simulink model "DiagramaDeBlocosDrone"  (R2014a)
settings: Solver=ode45  StartTime=0.0  StopTime=10.0  RelTol=1e-3
undefined symbols (not defined in the file): K
libraries: fuzblock x2
settings Model: Creator=ASAFE  LastModifiedBy=ASAFE

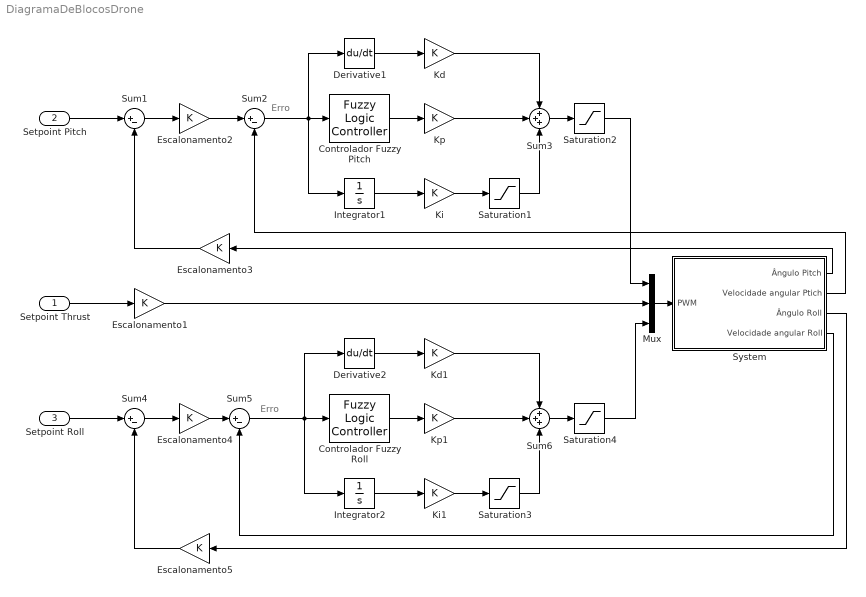
== system DiagramaDeBlocosDrone ==
  note: Erro
  note: Erro
  Setpoint Thrust : Inport
  Setpoint Pitch : Inport  Port=2
  Setpoint Roll : Inport  Port=3
  Controlador Fuzzy Pitch : fuzblock/Fuzzy Logic  Controller  fis=[]
  Controlador Fuzzy Roll : fuzblock/Fuzzy Logic  Controller  fis=[]
  Derivative1 : Derivative
  Derivative2 : Derivative
  Escalonamento{1..5} (5 alike) : Gain  Gain=K
  Integrator1 : Integrator
  Integrator2 : Integrator
  Kd : Gain  Gain=K
  Kd1 : Gain  Gain=K
  Ki : Gain  Gain=K
  Ki1 : Gain  Gain=K
  Kp : Gain  Gain=K
  Kp1 : Gain  Gain=K
  Mux : Mux  Inputs=3
  Saturation{1..4} (4 alike) : Saturate
  Sum{1..2,4..5} (4 alike) : Sum  Inputs=|+-
  Sum3 : Sum  Inputs=+++
  Sum6 : Sum  Inputs=+++
  System : Subsystem
  wires:
  Setpoint Pitch/1 -> Sum1/1
  Sum1/1 -> Escalonamento2/1
  Escalonamento2/1 -> Sum2/1
  Sum2/1 -> Derivative1/1, Integrator1/1, Controlador Fuzzy Pitch/1
  Derivative1/1 -> Kd/1
  Controlador Fuzzy Pitch/1 -> Kp/1
  Integrator1/1 -> Ki/1
  Ki/1 -> Saturation1/1
  Kp/1 -> Sum3/2
  Kd/1 -> Sum3/1
  Saturation1/1 -> Sum3/3
  Sum3/1 -> Saturation2/1
  Escalonamento3/1 -> Sum1/2
  Mux/1 -> System/1(PWM)
  Setpoint Thrust/1 -> Escalonamento1/1
  Setpoint Roll/1 -> Sum4/1
  Sum4/1 -> Escalonamento4/1
  Escalonamento4/1 -> Sum5/1
  Sum5/1 -> Integrator2/1, Derivative2/1, Controlador Fuzzy Roll/1
  Derivative2/1 -> Kd1/1
  Controlador Fuzzy Roll/1 -> Kp1/1
  Integrator2/1 -> Ki1/1
  Ki1/1 -> Saturation3/1
  Kp1/1 -> Sum6/2
  Kd1/1 -> Sum6/1
  Saturation3/1 -> Sum6/3
  Sum6/1 -> Saturation4/1
  Escalonamento5/1 -> Sum4/2
  Saturation4/1 -> Mux/3
  Escalonamento1/1 -> Mux/2
  Saturation2/1 -> Mux/1
  System/4(Velocidade angular Roll) -> Sum5/2
  System/1(Ângulo Pitch) -> Escalonamento3/1
  System/2(Velocidade angular Ptich) -> Sum2/2
  System/3(Ângulo Roll) -> Escalonamento5/1

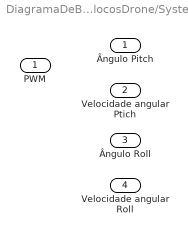
== system DiagramaDeBlocosDrone/System ==
  PWM : Inport
  Ângulo Pitch : Outport
  Velocidade angular Ptich : Outport  Port=2
  Ângulo Roll : Outport  Port=3
  Velocidade angular Roll : Outport  Port=4
